simulink model "ev_kart"  (R2019b)
settings: Solver=FixedStepDiscrete  StartTime=0.0  StopTime=inf  RelTol=1e-3  EnableMultiTasking=on
libraries: arduinolib x21, simulink x1
settings Model: EnablePacing=on  ExtModeTrigDuration=2  Creator=hirata  LastModifiedBy=k-abe
settings DataIOCC: LimitDataPoints=on  SaveFormat=Array  ReturnWorkspaceOutputs=off
settings OptimizationCC: EnhancedBackFolding=on  PassReuseOutputArgsThreshold=0  ExpressionDepthLimit=2147483647  MaxStackSize=64  OptimizeBlockOrder=speed  DifferentSizesBufferReuse=on  OptimizationCustomize=off
settings DebuggingCC: UnderspecifiedInitializationDetection=Classic  MergeDetectMultiDrivingBlocksExec=none  SolverPrmCheckMsg=warning  ParameterTunabilityLossMsg=error  FcnCallInpInsideContextMsg=warning  StateNameClashWarn=warning  SFUnexpectedBacktrackingDiag=warning  SFNoUnconditionalDefaultTransitionDiag=warning  SFExecutionAtInitializationDiag=none  ArithmeticOperatorsInVariantConditions=warning
settings HardwareCC: ProdBitPerInt=16  ProdBitPerPointer=16  ProdBitPerSizeT=16  ProdBitPerPtrDiffT=16  ProdLargestAtomicFloat=None  ProdWordSize=8  ProdHWDeviceType=Atmel->AVR  UseEmbeddedCoderFeatures=off  UseSimulinkCoderFeatures=off
settings ModelReferenceCC: PropagateSignalLabelsOutOfModel=off
settings SFSimCC: SimUseLocalCustomCode=off  MATLABDynamicMemAlloc=off  CustomCodeUndefinedFunction=UseInterfaceOnly
settings RTWCC: SystemTargetFile=ert.tlc  HardwareBoard=Arduino Mega 2560  TLCOptions=-aInlineSetEventsForThisBaseRateFcn=TLC_FALSE -aSuppressMultiTaskScheduler=TLC_FALSE -aRateBasedStepFcn=1  TemplateMakefile=ert_default_tmf  GenerateReport=on  RTWUseLocalCustomCode=off  Toolchain=Arduino AVR  BuildConfiguration=Faster Runs  LaunchReport=on
settings CodeAppCC: ForceParamTrailComments=on  OperatorAnnotations=on
settings ERTTargetCC: ERTCustomFileBanners=off  SupportContinuousTime=on  SupportNonInlinedSFcns=on  RemoveResetFunc=off  SupportVariableSizeSignals=on  ModelStepFunctionPrototypeControlCompliant=off
settings ConfigComp: CovMetricSettings=dw  CovHtmlReporting=on  CovSaveCumulativeToWorkspaceVar=on  CovSaveSingleToWorkspaceVar=on  CovExternalEMLEnable=off

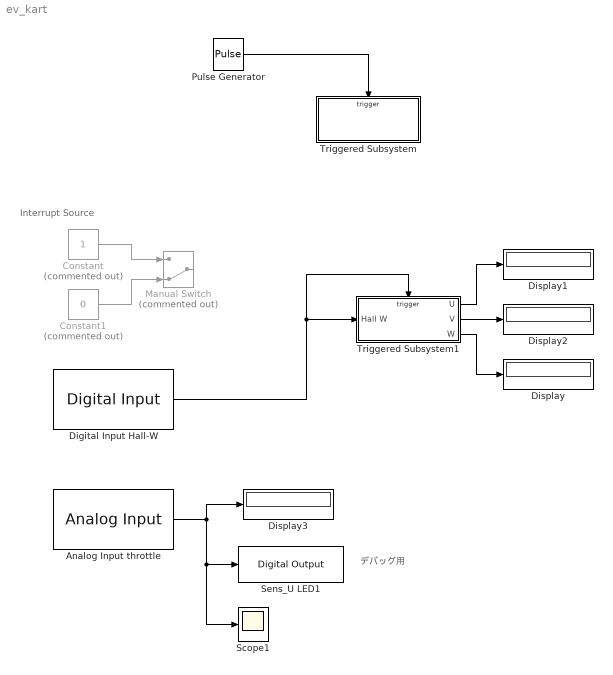
== system ev_kart ==
  note: デバッグ用
  note: Interrupt Source
  Analog Input throttle : arduinolib/Analog Input  pinNumber=0  ReadResultsOnly=off  ConversionTriggerSource=Software  ExternalTriggerType=uint32(0)  OutputDataType=uint16  EnableConversionCompleteNotify=off  EnableOuputStatus=off  SampleTime=-1  blockPlatform=arduino
  Constant : Constant  Commented=on  OutDataTypeStr=boolean  SampleTime=0.1
  Constant1 : Constant  Commented=on  Value=0  OutDataTypeStr=boolean  SampleTime=0.1
  Digital Input Hall-W : arduinolib/Digital Input  pinNumber=21  SampleTime=1/50  blockPlatform=arduino
      settings: SourceProductName=Simulink Support Package for Arduino Hardware
  Display{,1..3} (4 alike) : Display
  Manual Switch : ManualSwitch  Commented=on  CurrentSetting=0
  Pulse Generator : DiscretePulseGenerator  PulseType=Time based  Period=1  PulseWidth=50
  Scope1 : Scope
  Sens_U LED1 : arduinolib/Digital Output  pinNumber=23  blockPlatform=arduino
  Triggered Subsystem : Subsystem  TreatAsAtomicUnit=on
  Triggered Subsystem1 : Subsystem  TreatAsAtomicUnit=on
  wires:
  Pulse Generator/1 -> Triggered Subsystem/Trigger
  Constant1/1 -> Manual Switch/2
  Constant/1 -> Manual Switch/1
  Triggered Subsystem1/3(W) -> Display/1
  Triggered Subsystem1/1(U) -> Display1/1
  Triggered Subsystem1/2(V) -> Display2/1
  Digital Input Hall-W/1 -> Triggered Subsystem1/Trigger, Triggered Subsystem1/1(Hall W)
  Analog Input throttle/1 -> Scope1/1, Sens_U LED1/1, Display3/1

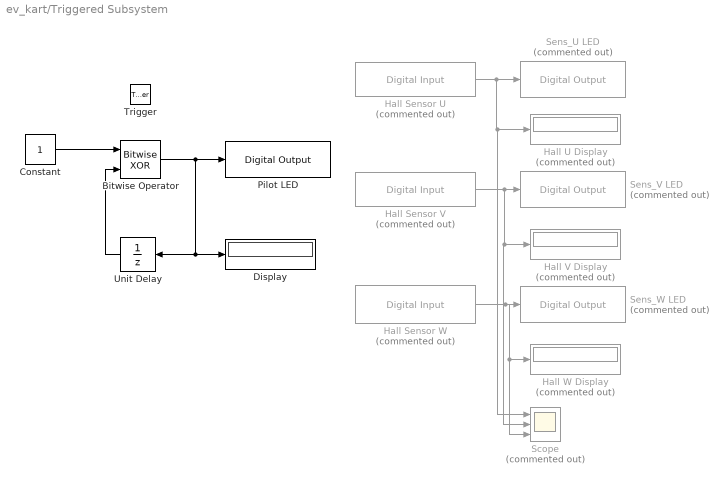
== system ev_kart/Triggered Subsystem ==
  Trigger : TriggerPort  VariantControl=Variant
  Bitwise Operator : simulink/Logic and Bit Operations/Bitwise Operator  logicop=XOR  UseBitMask=off  NumInputPorts=2  BitMask=bin2dec('11011001')  BitMaskRealWorld=Stored Integer
  Constant : Constant  OutDataTypeStr=uint8
  Display : Display
  Hall Sensor U : arduinolib/Digital Input  Commented=on  pinNumber=19  SampleTime=-1  blockPlatform=arduino
      settings: SourceProductName=Simulink Support Package for Arduino Hardware
  Hall Sensor V : arduinolib/Digital Input  Commented=on  pinNumber=20  SampleTime=-1  blockPlatform=arduino
      settings: SourceProductName=Simulink Support Package for Arduino Hardware
  Hall Sensor W : arduinolib/Digital Input  Commented=on  pinNumber=21  SampleTime=-1  blockPlatform=arduino
      settings: SourceProductName=Simulink Support Package for Arduino Hardware
  Hall U Display : Display  Commented=on
  Hall V Display : Display  Commented=on
  Hall W Display : Display  Commented=on
  Pilot LED : arduinolib/Digital Output  pinNumber=13  blockPlatform=arduino
  Scope : Scope  Commented=on  NumInputPorts=3
  Sens_U LED : arduinolib/Digital Output  Commented=on  pinNumber=23  blockPlatform=arduino
  Sens_V LED : arduinolib/Digital Output  Commented=on  pinNumber=25  blockPlatform=arduino
  Sens_W LED : arduinolib/Digital Output  Commented=on  pinNumber=27  blockPlatform=arduino
  Unit Delay : UnitDelay  SampleTime=-1  HasFrameUpgradeWarning=on
  wires:
  Constant/1 -> Bitwise Operator/1
  Bitwise Operator/1 -> Pilot LED/1, Unit Delay/1, Display/1
  Unit Delay/1 -> Bitwise Operator/2
  Hall Sensor W/1 -> Scope/3, Hall W Display/1, Sens_W LED/1
  Hall Sensor V/1 -> Hall V Display/1, Scope/2, Sens_V LED/1
  Hall Sensor U/1 -> Scope/1, Hall U Display/1, Sens_U LED/1

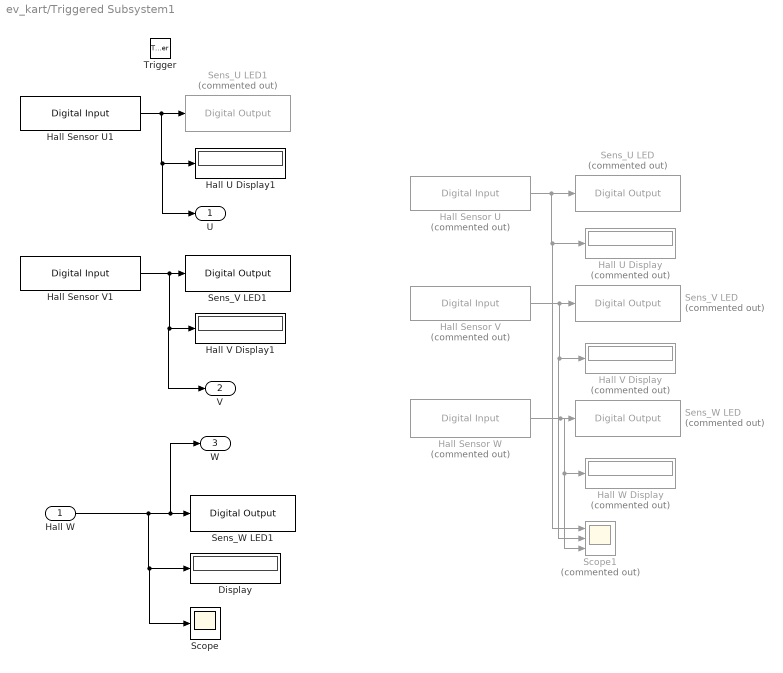
== system ev_kart/Triggered Subsystem1 ==
  Hall W : Inport
  Trigger : TriggerPort  TriggerType=either  VariantControl=Variant
  Display : Display
  Hall Sensor U : arduinolib/Digital Input  Commented=on  pinNumber=19  SampleTime=-1  blockPlatform=arduino
      settings: SourceProductName=Simulink Support Package for Arduino Hardware
  Hall Sensor U1 : arduinolib/Digital Input  pinNumber=19  SampleTime=-1  blockPlatform=arduino
      settings: SourceProductName=Simulink Support Package for Arduino Hardware
  Hall Sensor V : arduinolib/Digital Input  Commented=on  pinNumber=20  SampleTime=-1  blockPlatform=arduino
      settings: SourceProductName=Simulink Support Package for Arduino Hardware
  Hall Sensor V1 : arduinolib/Digital Input  pinNumber=20  SampleTime=-1  blockPlatform=arduino
      settings: SourceProductName=Simulink Support Package for Arduino Hardware
  Hall Sensor W : arduinolib/Digital Input  Commented=on  pinNumber=21  SampleTime=-1  blockPlatform=arduino
      settings: SourceProductName=Simulink Support Package for Arduino Hardware
  Hall U Display : Display  Commented=on
  Hall U Display1 : Display
  Hall V Display : Display  Commented=on
  Hall V Display1 : Display
  Hall W Display : Display  Commented=on
  Scope : Scope
  Scope1 : Scope  Commented=on  NumInputPorts=3
  Sens_U LED : arduinolib/Digital Output  Commented=on  pinNumber=23  blockPlatform=arduino
  Sens_U LED1 : arduinolib/Digital Output  Commented=on  pinNumber=23  blockPlatform=arduino
  Sens_V LED : arduinolib/Digital Output  Commented=on  pinNumber=25  blockPlatform=arduino
  Sens_V LED1 : arduinolib/Digital Output  pinNumber=25  blockPlatform=arduino
  Sens_W LED : arduinolib/Digital Output  Commented=on  pinNumber=27  blockPlatform=arduino
  Sens_W LED1 : arduinolib/Digital Output  pinNumber=27  blockPlatform=arduino
  U : Outport
  V : Outport  Port=2
  W : Outport  Port=3
  wires:
  Hall W/1 -> W/1, Sens_W LED1/1, Scope/1, Display/1
  Hall Sensor V/1 -> Hall V Display/1, Scope1/2, Sens_V LED/1
  Hall Sensor W/1 -> Scope1/3, Hall W Display/1, Sens_W LED/1
  Hall Sensor U/1 -> Scope1/1, Hall U Display/1, Sens_U LED/1
  Hall Sensor U1/1 -> U/1, Hall U Display1/1, Sens_U LED1/1
  Hall Sensor V1/1 -> Hall V Display1/1, V/1, Sens_V LED1/1
